simulink model "AVR"  (R2020a)
settings: Solver=VariableStepAuto  StartTime=0.0  StopTime=7.5  FixedStep=0.005  RelTol=1e-4
libraries: fmu_me_lib x1
settings Model: Creator=meagh

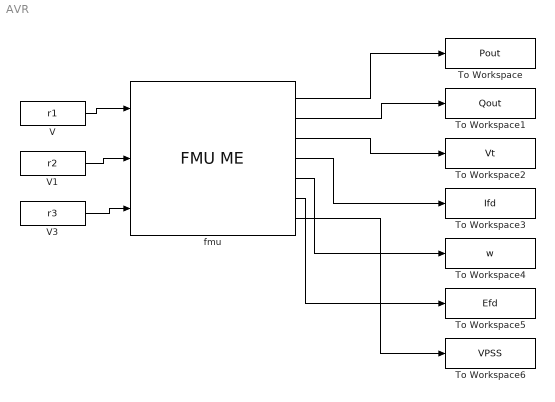
== system AVR ==
  To Workspace : ToWorkspace  VariableName=Pout  SaveFormat=Timeseries  SampleTime=0.005
  To Workspace1 : ToWorkspace  VariableName=Qout  SaveFormat=Timeseries  SampleTime=0.005
  To Workspace2 : ToWorkspace  VariableName=Vt  SaveFormat=Timeseries  SampleTime=0.005
  To Workspace3 : ToWorkspace  VariableName=Ifd  SaveFormat=Timeseries  SampleTime=0.005
  To Workspace4 : ToWorkspace  VariableName=w  SaveFormat=Timeseries  SampleTime=0.005
  To Workspace5 : ToWorkspace  VariableName=Efd  SaveFormat=Timeseries  SampleTime=0.005
  To Workspace6 : ToWorkspace  VariableName=VPSS  SaveFormat=Timeseries  SampleTime=0.005
  V : FromWorkspace  VariableName=r1
  V1 : FromWorkspace  VariableName=r2
  V3 : FromWorkspace  VariableName=r3
  fmu : fmu_me_lib/FMU ME  Description=Simulates an FMU for Model Exchange 1.0 or Model Exchange 2.0.  dummy=0
  wires:
  V/1 -> fmu/1
  V1/1 -> fmu/2
  fmu/1 -> To Workspace/1
  V3/1 -> fmu/3
  fmu/2 -> To Workspace1/1
  fmu/3 -> To Workspace2/1
  fmu/4 -> To Workspace3/1
  fmu/5 -> To Workspace4/1
  fmu/6 -> To Workspace5/1
  fmu/7 -> To Workspace6/1
